simulink model "ac"  (R2024b)
settings: Solver=VariableStepAuto  StartTime=0.0  StopTime=inf  RelTol=1e-3
settings Model: Creator=HP  LastModifiedBy=HP

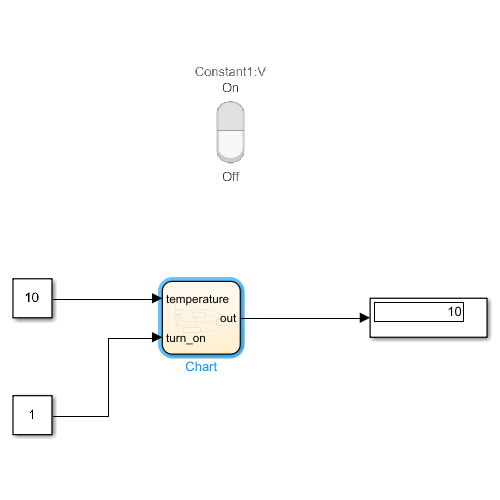
[thumbnail: Simulink's stored preview of the top-level diagram]
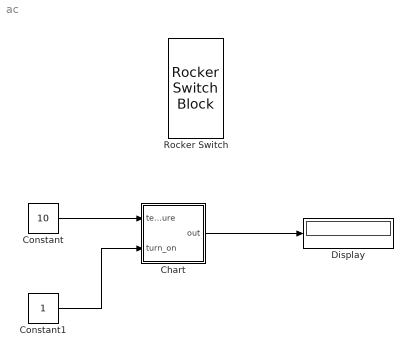
== system ac ==
  Chart : Stateflow chart  TreatAsAtomicUnit=on
  Constant : Constant  Value=10
  Constant1 : Constant
  Display : Display
  Rocker Switch : RockerSwitchBlock
      settings: Values={{'Off', 'On'}, [0 1]}
  wires:
  Chart/1(out) -> Display/1
  Constant/1 -> Chart/1(temperature)
  Constant1/1 -> Chart/2(turn_on)

== stateflow chart ac/Chart ==
  state on_off
    out=0
  state steady
    out=heat_temp
  state heat_on
    heat_temp=heat_temp+1
    out=heat_temp
  state cooler_on
    heat_temp=heat_temp-1
    out=heat_temp
  (default) -> on_off : {heat_temp=0}
  on_off -> heat_on [order 1] : [turn_on==1&&heat_temp<temperature]
  cooler_on -> on_off [order 3] : [turn_on==0]
  on_off -> cooler_on [order 2] : [turn_on==1&&...
      | heat_temp>temperature]
  heat_on -> on_off [order 2] : [turn_on==0]
  steady -> on_off : [heat_temp~=temperature||...
      | turn_on==0]
  heat_on -> steady [order 3] : [heat_temp==temperature]
  cooler_on -> steady [order 1] : [heat_temp==temperature]
  cooler_on -> heat_on [order 2] : [heat_temp<temperature]
  heat_on -> cooler_on [order 1] : [heat_temp>temperature]
  data: temperature input; out output [-30..40] =0; turn_on input; heat_temp local [-30..40] =0
